simulink model "parrot_vision_ext_mode_imfindcircles"  (R2021a)
settings: Solver=FixedStepAuto  StartTime=0.0  StopTime=100  RelTol=1e-3  EnableMultiTasking=on
InitFcn:
  | load('BusDefinitions.mat')
  | codertarget.parrot.internal.checkImageBlocks(gcs)
undefined symbols (not defined in the file): BINARIZATION_THRESHOLD, codertarget, G_B_GAIN, Rmax, Rmin, Ts
libraries: parrotlib x1
settings Model: SimulationMode=external  ExtModeTrigDuration=80  Creator=The MathWorks, Inc.  LastModifiedBy=s2130866
settings SolverCC: AlgebraicLoopSolver=TrustRegion  PositivePriorityOrder=on
settings DataIOCC: ReturnWorkspaceOutputs=off
settings OptimizationCC: PassReuseOutputArgsThreshold=0  MaxStackSize=64
settings DebuggingCC: ParameterTunabilityLossMsg=error  PregeneratedLibrarySubsystemCodeDiagnostic=none  SFMachineParentedDataDiag=warning  ArithmeticOperatorsInVariantConditions=warning
settings HardwareCC: ProdBitPerPointer=32  ProdBitPerSizeT=32  ProdBitPerPtrDiffT=32  ProdLargestAtomicInteger=Long  ProdWordSize=32  ProdHWDeviceType=ARM Compatible->ARM 9  UseEmbeddedCoderFeatures=off  UseSimulinkCoderFeatures=off
settings SFSimCC: SimUseLocalCustomCode=off  MATLABDynamicMemAlloc=off  CustomCodeUndefinedFunction=UseInterfaceOnly
settings RTWCC: SystemTargetFile=ert.tlc  HardwareBoard=PARROT Mambo  TemplateMakefile=ert_default_tmf  GenerateReport=on  RTWUseLocalCustomCode=off  Toolchain=Sourcery G++ Lite GNU Toolchain for Drones  LaunchReport=on
settings CodeAppCC: ForceParamTrailComments=on  OperatorAnnotations=on  StateflowObjectComments=on
settings ERTTargetCC: ERTCustomFileBanners=off  SupportContinuousTime=on  SupportNonInlinedSFcns=on  RemoveResetFunc=off  ModelStepFunctionPrototypeControlCompliant=off

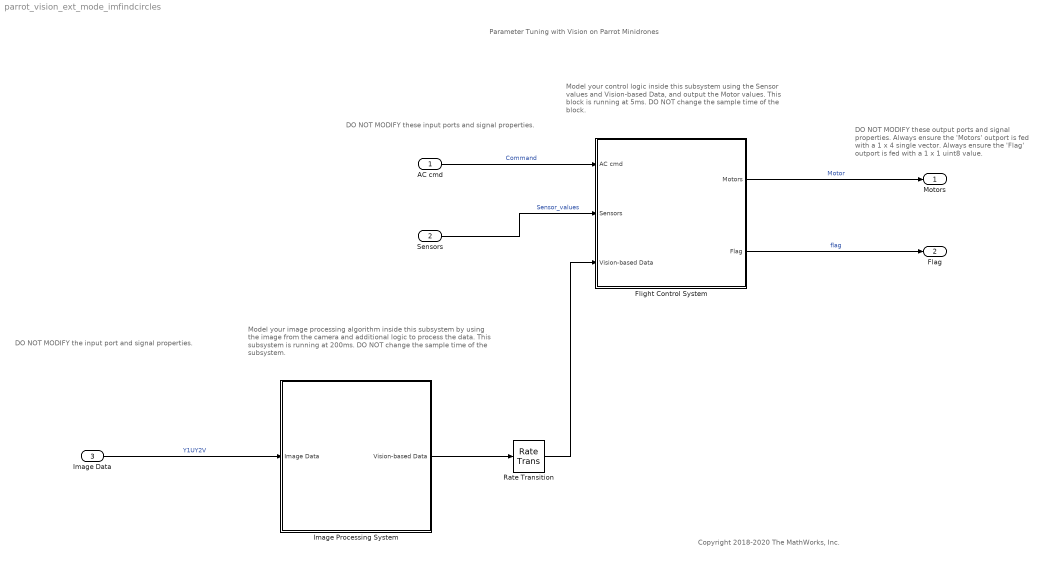
== system parrot_vision_ext_mode_imfindcircles ==
  note: Model your control logic inside this subsystem
      | using the Sensor values and Vision-based Data,
      | and output the Motor values.
      | This block is running at 5ms.
      | DO NOT change the sample time of the block.
  note: DO NOT MODIFY these output ports
      | and signal properties.
      |
      |
      |
      |
      |
      | Always ensure the 'Motors' outport
      | is fed with a 1 x 4 single vector.
      |
      |
      |
      |
      |
      | Always ensure the 'Flag' outport is
      | fed with a 1 x 1 uint8 value.
  note: DO NOT MODIFY these input
      | ports and signal properties.
  note: Copyright 2018-2020 The MathWorks, Inc.
  note: Parameter Tuning with Vision on Parrot Minidrones
  note: DO NOT MODIFY the input port and
      | signal properties.
  note: Model your image processing algorithm inside this
      | subsystem by using the image from the camera
      | and additional logic to process the data.
      | This subsystem is running at 200ms.
      | DO NOT change the sample time of the subsystem.
  AC cmd : Inport  OutDataTypeStr=Bus: CommandBus  BusOutputAsStruct=on
  Sensors : Inport  Port=2  OutDataTypeStr=Bus: SensorsBus  BusOutputAsStruct=on
  Image Data : Inport  Tag=IP_IN  InitFcn=codertarget.parrot.internal.inportCallback(gcb);  Port=3  OutDataTypeStr=uint8  PortDimensions=[4 9600]  BusOutputAsStruct=on
  Flight Control System : Subsystem  InitFcn=codertarget.parrot.internal.fcsSubsystemCallback(gcb);  TreatAsAtomicUnit=on  SystemSampleTime=Ts
  Image Processing System : Subsystem  Tag=IP_SUB  InitFcn=codertarget.parrot.internal.ipSubsystemCallback(gcb);  TreatAsAtomicUnit=on  SystemSampleTime=40*Ts  RTWFcnName=ImageFunction
      settings: RTWSystemCode=Inline  RTWFcnNameOpts=User specified
  Rate Transition : RateTransition  Deterministic=off
  Motors : Outport  OutDataTypeStr=single  PortDimensions=[1 4]  VectorParamsAs1DForOutWhenUnconnected=off
  Flag : Outport  Port=2  OutDataTypeStr=uint8  PortDimensions=1  VectorParamsAs1DForOutWhenUnconnected=off
  wires:
  Flight Control System/1(Motors) -> Motors/1  "Motor"
  AC cmd/1 -> Flight Control System/1(AC cmd)  "Command"
  Sensors/1 -> Flight Control System/2(Sensors)  "Sensor_values"
  Flight Control System/2(Flag) -> Flag/1  "flag"
  Image Data/1 -> Image Processing System/1(Image Data)  "Y1UY2V"
  Rate Transition/1 -> Flight Control System/3(" Vision-based Data")
  Image Processing System/1(" Vision-based Data") -> Rate Transition/1

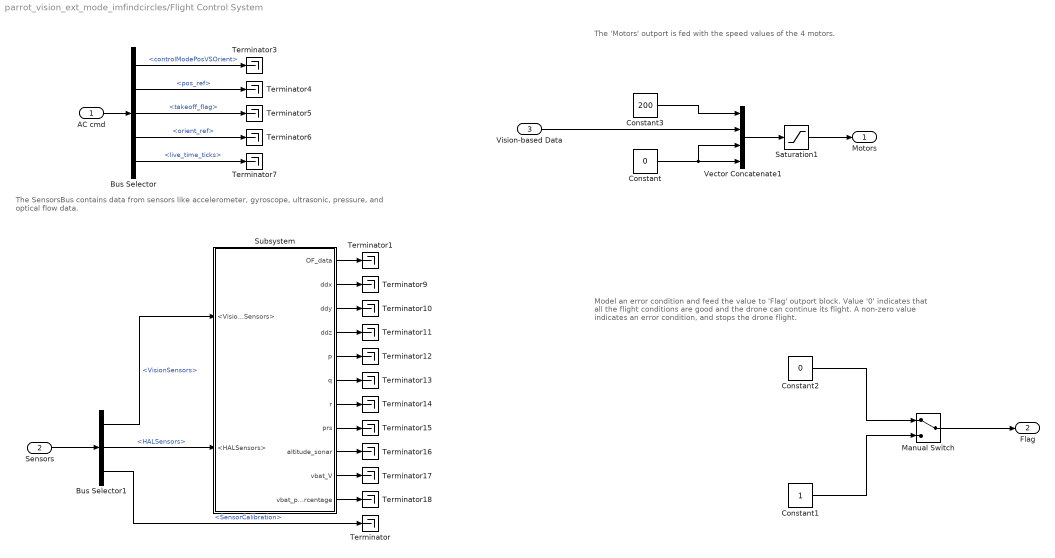
== system parrot_vision_ext_mode_imfindcircles/Flight Control System ==
  note: The 'Motors' outport is fed with the speed values of the 4 motors.
  note: Model an error condition and feed the value to 'Flag' outport block.
      | Value '0' indicates that all the flight conditions are good and the drone
      | can continue its flight.
      | A non-zero value indicates an error condition, and stops the drone
      | flight.
  note: The SensorsBus contains data from sensors like
      | accelerometer, gyroscope, ultrasonic, pressure,
      | and optical flow data.
  AC cmd : Inport
  Sensors : Inport  Port=2
  " Vision-based Data" : Inport  Port=3
  Bus Selector : BusSelector  OutputSignals=controlModePosVSOrient,pos_ref,takeoff_flag,orient_ref,live_time_ticks
  Bus Selector1 : BusSelector  OutputSignals=VisionSensors,HALSensors,SensorCalibration
  Constant : Constant  Value=0
  Constant1 : Constant  OutDataTypeStr=uint8
  Constant2 : Constant  Value=0  OutDataTypeStr=uint8
  Constant3 : Constant  Value=200
  Manual Switch : ManualSwitch
  Saturation1 : Saturate  UpperLimit=500  LowerLimit=0  OutDataTypeStr=single
  Subsystem : Subsystem
  Terminator{,1,3..7,9..18} (17 alike) : Terminator
  Vector Concatenate1 : Concatenate  NumInputs=4
  Motors : Outport  VectorParamsAs1DForOutWhenUnconnected=off
  Flag : Outport  Port=2  VectorParamsAs1DForOutWhenUnconnected=off
  wires:
  AC cmd/1 -> Bus Selector/1
  Sensors/1 -> Bus Selector1/1
  Bus Selector/1 -> Terminator3/1  "<controlModePosVSOrient>"
  Bus Selector/2 -> Terminator4/1  "<pos_ref>"
  Bus Selector/3 -> Terminator5/1  "<takeoff_flag>"
  Bus Selector/4 -> Terminator6/1  "<orient_ref>"
  Bus Selector/5 -> Terminator7/1  "<live_time_ticks>"
  Manual Switch/1 -> Flag/1
  Constant2/1 -> Manual Switch/1
  Constant1/1 -> Manual Switch/2
  Vector Concatenate1/1 -> Saturation1/1
  Saturation1/1 -> Motors/1
  Bus Selector1/1 -> Subsystem/1(<VisionSensors>)  "<VisionSensors>"
  Bus Selector1/2 -> Subsystem/2(<HALSensors>)  "<HALSensors>"
  Bus Selector1/3 -> Terminator/1  "<SensorCalibration>"
  Subsystem/1(OF_data) -> Terminator1/1
  Subsystem/2(ddx) -> Terminator9/1
  Subsystem/3(ddy) -> Terminator10/1
  Subsystem/4(ddz) -> Terminator11/1
  Subsystem/5(p) -> Terminator12/1
  Subsystem/7(r) -> Terminator14/1
  Subsystem/8(prs) -> Terminator15/1
  Subsystem/9(altitude_sonar) -> Terminator16/1
  Subsystem/10(vbat_V) -> Terminator17/1
  Subsystem/11(vbat_percentage) -> Terminator18/1
  Subsystem/6(q) -> Terminator13/1
  Constant/1 -> Vector Concatenate1/3, Vector Concatenate1/4
  " Vision-based Data"/1 -> Vector Concatenate1/2
  Constant3/1 -> Vector Concatenate1/1

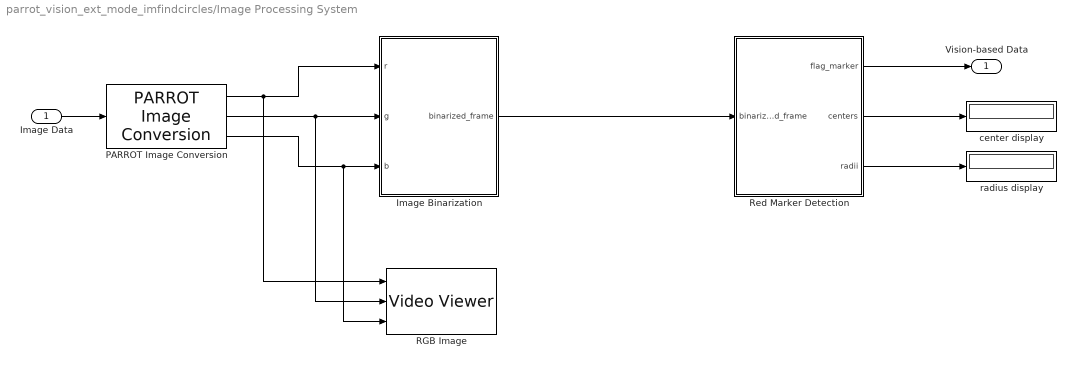
== system parrot_vision_ext_mode_imfindcircles/Image Processing System ==
  Image Data : Inport
  Image Binarization : MATLAB Function  TreatAsAtomicUnit=on
  "PARROT Image Conversion " : parrotlib/PARROT Image Conversion  Tag=IP_FORMAT  ImageFormat=RGB  R=on  Y=on  G=on  U=on  B=on  V=on
  RGB Image : VideoViewer  imagePorts=separate color signals  FigPos=[728.333333333333 670.666666666667 485.333333333333 388]
  Red Marker Detection : MATLAB Function  TreatAsAtomicUnit=on
  center display : Display
  radius display : Display
  " Vision-based Data" : Outport  VectorParamsAs1DForOutWhenUnconnected=off
  wires:
  Image Data/1 -> "PARROT Image Conversion "/1
  Image Binarization/1(binarized_frame) -> Red Marker Detection/1(binarized_frame)
  Red Marker Detection/1(flag_marker) -> " Vision-based Data"/1
  Red Marker Detection/2(centers) -> center display/1
  "PARROT Image Conversion "/1 -> RGB Image/1, Image Binarization/1(r)
  "PARROT Image Conversion "/2 -> RGB Image/2, Image Binarization/2(g)
  "PARROT Image Conversion "/3 -> RGB Image/3, Image Binarization/3(b)
  Red Marker Detection/3(radii) -> radius display/1

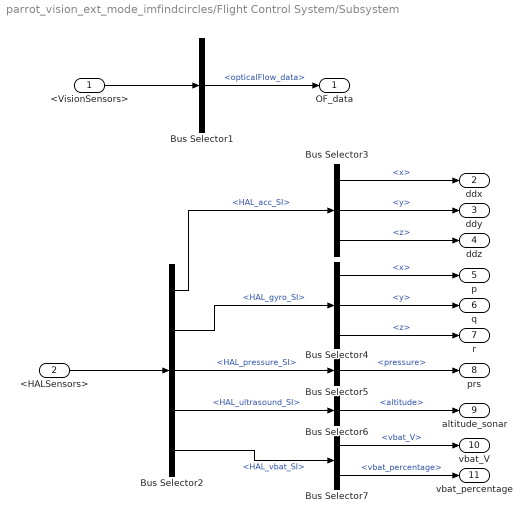
== system parrot_vision_ext_mode_imfindcircles/Flight Control System/Subsystem ==
  <VisionSensors> : Inport
  <HALSensors> : Inport  Port=2
  Bus Selector1 : BusSelector  OutputSignals=opticalFlow_data
  Bus Selector2 : BusSelector  OutputSignals=HAL_acc_SI,HAL_gyro_SI,HAL_pressure_SI,HAL_ultrasound_SI,HAL_vbat_SI
  Bus Selector3 : BusSelector  OutputSignals=x,y,z
  Bus Selector4 : BusSelector  OutputSignals=x,y,z
  Bus Selector5 : BusSelector  OutputSignals=pressure
  Bus Selector6 : BusSelector  OutputSignals=altitude
  Bus Selector7 : BusSelector  OutputSignals=vbat_V,vbat_percentage
  OF_data : Outport  VectorParamsAs1DForOutWhenUnconnected=off
  ddx : Outport  Port=2  VectorParamsAs1DForOutWhenUnconnected=off
  ddy : Outport  Port=3  VectorParamsAs1DForOutWhenUnconnected=off
  ddz : Outport  Port=4  VectorParamsAs1DForOutWhenUnconnected=off
  p : Outport  Port=5  VectorParamsAs1DForOutWhenUnconnected=off
  q : Outport  Port=6  VectorParamsAs1DForOutWhenUnconnected=off
  r : Outport  Port=7  VectorParamsAs1DForOutWhenUnconnected=off
  prs : Outport  Port=8  VectorParamsAs1DForOutWhenUnconnected=off
  altitude_sonar : Outport  Port=9  VectorParamsAs1DForOutWhenUnconnected=off
  vbat_V : Outport  Port=10  VectorParamsAs1DForOutWhenUnconnected=off
  vbat_percentage : Outport  Port=11  VectorParamsAs1DForOutWhenUnconnected=off
  wires:
  <VisionSensors>/1 -> Bus Selector1/1
  <HALSensors>/1 -> Bus Selector2/1
  Bus Selector1/1 -> OF_data/1  "<opticalFlow_data>"
  Bus Selector2/1 -> Bus Selector3/1  "<HAL_acc_SI>"
  Bus Selector2/2 -> Bus Selector4/1  "<HAL_gyro_SI>"
  Bus Selector2/3 -> Bus Selector5/1  "<HAL_pressure_SI>"
  Bus Selector2/4 -> Bus Selector6/1  "<HAL_ultrasound_SI>"
  Bus Selector2/5 -> Bus Selector7/1  "<HAL_vbat_SI>"
  Bus Selector3/1 -> ddx/1  "<x>"
  Bus Selector3/2 -> ddy/1  "<y>"
  Bus Selector3/3 -> ddz/1  "<z>"
  Bus Selector4/2 -> q/1  "<y>"
  Bus Selector4/1 -> p/1  "<x>"
  Bus Selector4/3 -> r/1  "<z>"
  Bus Selector5/1 -> prs/1  "<pressure>"
  Bus Selector6/1 -> altitude_sonar/1  "<altitude>"
  Bus Selector7/1 -> vbat_V/1  "<vbat_V>"
  Bus Selector7/2 -> vbat_percentage/1  "<vbat_percentage>"

== matlab function parrot_vision_ext_mode_imfindcircles/Image Processing System/Image Binarization ==
  data: r input; binarized_frame output; g input; b input; G_B_GAIN parameter; BINARIZATION_THRESHOLD parameter
function binarized_frame = binarizer(r, g, b,G_B_GAIN, BINARIZATION_THRESHOLD)
% The MATLAB function computes a binarized frame starting from a frame 
% expressed in the RGB file format. 
%
% Inputs:
% - r: Red channel frame
% - g: Green channel frame
% - b: Blue channel frame
%
% Output:
% - binarze_frame: the binarized frame
%
% Parameters:
% - G_B_GAIN: used to reduce the amount of green and blue colors inside the frame
% - BINARIZER_THRESHOLD: threshold to detect only the track inside the frame 

frame= r - (g/G_B_GAIN) - (b/G_B_GAIN);

binarized_frame = frame >= BINARIZATION_THRESHOLD;

end

== matlab function parrot_vision_ext_mode_imfindcircles/Image Processing System/Red Marker Detection ==
  data: binarized_frame input; flag_marker output; centers output; radii output; Rmin parameter; Rmax parameter
function [flag_marker, centers, radii] = Markerdetector(binarized_frame,Rmin, Rmax)
% % The MATLAB Function finds the circle in the image captured by the
% % downward camera and returns the circle's center and radii. 
% 
% Inputs:
% binarized_frame: the binary form of the image
% 
% Outputs:
% flag_marker: flag variable of detecting the drone
% 
% Parameters:
% Rmin: the minimum seachering radius range
% Rmax: the maximum searchering radius range

%shows the image
%imshow(binarized_frame)
%The argument'two stages' specifies the circular hough transform method
flag_marker = 0;
centers = zeros(1,2);
radii = 0;
[centers,radii] = imfindcircles(binarized_frame,[Rmin Rmax],'ObjectPolarity','bright', 'Sensitivity',0.97,'Method','twostage');
%h = viscircles(centers,radii);
%center_str = sprintf('(%2.2f,%2.2f)',centers(1),centers(2));
%text(centers(1),centers(2),center_str,'Color','g','FontSize',8,'FontWeight','bold')

%check if the centers and radii variable are empty, determining whether
%circle is detected
if radii == 0
    flag_marker = 0;
else
    flag_marker = 1;
end
end
